simulink model "MassSpringDamper_Project3"  (R2016b)
settings: Solver=VariableStepAuto  StartTime=0.0  StopTime=10.0  RelTol=1e-3
values from neighbouring files (symbols this model uses):
  b = 10    [MPD_TimeDomain.m]
  F = 1    [MPD_TimeDomain.m]
  k = 20    [MPD_TimeDomain.m]
  M = 1    [MPD_TimeDomain.m]
settings Model: Creator=1026691  LastModifiedBy=1026691

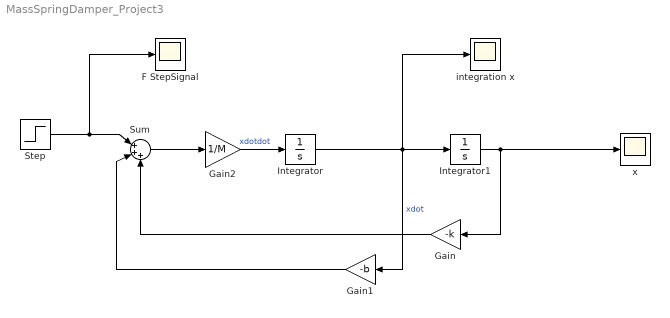
== system MassSpringDamper_Project3 ==
  "F StepSignal " : Scope
  Gain : Gain  Gain=-k
  Gain1 : Gain  Gain=-b
  Gain2 : Gain  Gain=1/M
  Integrator : Integrator
  Integrator1 : Integrator
  Step : Step  After=F  SampleTime=0
  Sum : Sum  Inputs=|+++
  integration x : Scope
  x : Scope
  wires:
  Integrator/1 -> integration x/1, Gain1/1, Integrator1/1  "xdot"
  Gain2/1 -> Integrator/1  "xdotdot"
  Step/1 -> "F StepSignal "/1, Sum/1
  Gain1/1 -> Sum/2
  Gain/1 -> Sum/3
  Integrator1/1 -> x/1, Gain/1
  Sum/1 -> Gain2/1
